simulink model "Pendulum_ViscousDamping"  (R2023b)
settings: Solver=VariableStepAuto  StartTime=0.0  StopTime=10  MaxStep=0.01  RelTol=1e-3
settings Model: Creator=Shubhada  LastModifiedBy=siva kumar
settings SolverCC: AlgebraicLoopSolver=TrustRegion
settings DataIOCC: ExternalInput=data  SaveFormat=Array  DSMLogging=off  ReturnWorkspaceOutputs=off
settings DebuggingCC: UnconnectedInputMsg=warning  UnconnectedOutputMsg=warning  UnconnectedLineMsg=warning
settings ModelReferenceCC: EnableRefExpFcnMdlSchedulingChecks=on
settings SFSimCC: CustomCodeUndefinedFunction=UseInterfaceOnly

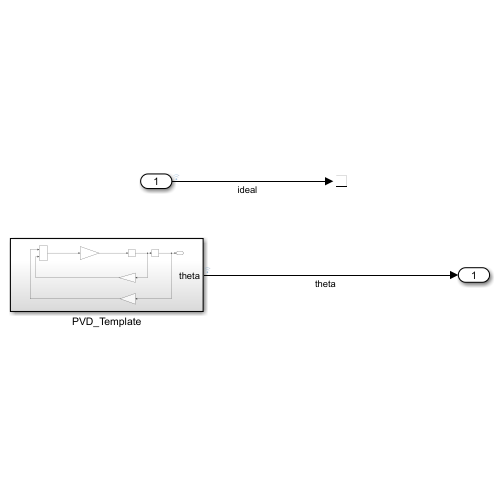
[thumbnail: Simulink's stored preview of the top-level diagram]
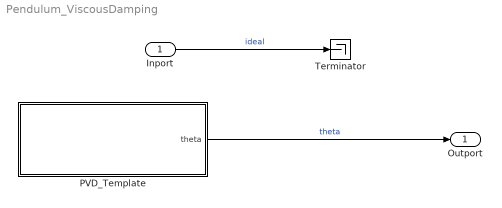
== system Pendulum_ViscousDamping ==
  Inport : Inport
  PVD_Template : Subsystem
  Terminator : Terminator
  Outport : Outport
  wires:
  PVD_Template/1(theta) -> Outport/1  "theta"
  Inport/1 -> Terminator/1  "ideal"

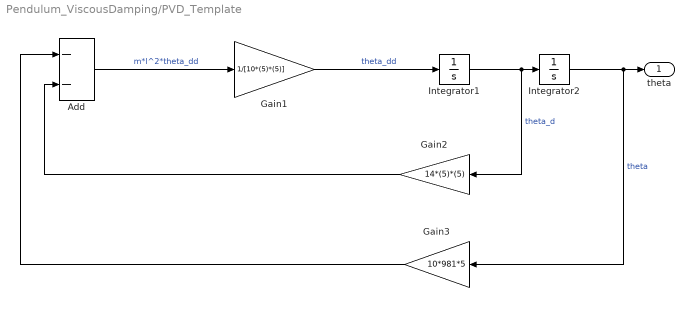
== system Pendulum_ViscousDamping/PVD_Template ==
  Add : Sum  Inputs=--
  Gain1 : Gain  Gain=1/[10*(5)*(5)]
  Gain2 : Gain  Gain=14*(5)*(5)
  Gain3 : Gain  Gain=10*981*5
  Integrator1 : Integrator
  Integrator2 : Integrator  InitialCondition=1.57
  theta : Outport
  wires:
  Add/1 -> Gain1/1  "m*l^2*theta_dd"
  Gain1/1 -> Integrator1/1  "theta_dd"
  Integrator1/1 -> Gain2/1, Integrator2/1  "theta_d"
  Integrator2/1 -> Gain3/1, theta/1  "theta"
  Gain2/1 -> Add/2
  Gain3/1 -> Add/1
